simulink model "GFL_phasejump"  (R2022a)
settings: Solver=FixedStepAuto  StartTime=0.0  StopTime=t_end+t_sim_start  FixedStep=Ts  RelTol=1e-3
undefined symbols (not defined in the file or in its folder): Cf, dc_ref, DiscIntNeverNeededParam, dt, Id0, Id_limit, initial, Iq0, ki_pll, ki_v_dc, kp_pll, kp_v_dc, Lc, Lf, Lg1, Lg11, Lgg, m_v, phasejum, Rf, Rg1, Rg11, Rgg, Sbase, t0, t0_jump, t_sim_start, tc, Ts, v_sag, Vac_ref, Vbase, Vdc_ref, w_i_GFL, w_limit, w_pll, w_tau, w_tvc, Wbase, Y_dc, Zbase
libraries: spsVoltageMeasurementLib x41, spsCurrentMeasurementLib x36, spsThreePhaseSeriesRLCBranchLib x14, spsControlledVoltageSourceLib x12, spsSeriesRLCBranchLib x8, spsControlledCurrentSourceLib x4, spsIdealSwitchLib x3, spsThreePhaseBreakerLib x2, spsDCVoltageSourceLib x1, spsThreePhaseParallelRLCBranchLib x1, spsThreePhaseFaultLib x1, spspowerguiLib x1
(part 1 of 3)
settings Model: Creator=admin_user  LastModifiedBy=yz7521
settings SolverCC: AlgebraicLoopSolver=TrustRegion
settings DataIOCC: ReturnWorkspaceOutputs=off
settings DebuggingCC: SFMachineParentedDataDiag=warning
settings RTWCC: DLArmComputeVersion=19.05

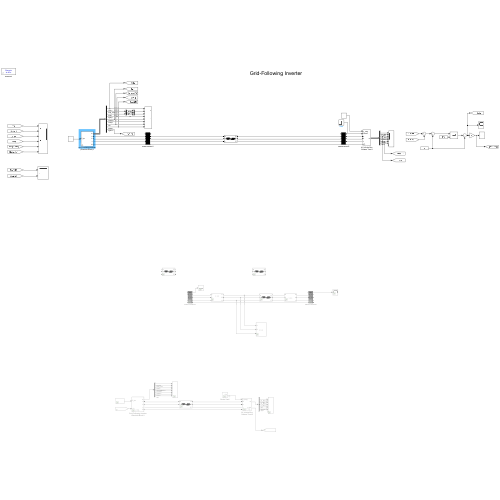
[thumbnail: Simulink's stored preview of the top-level diagram]
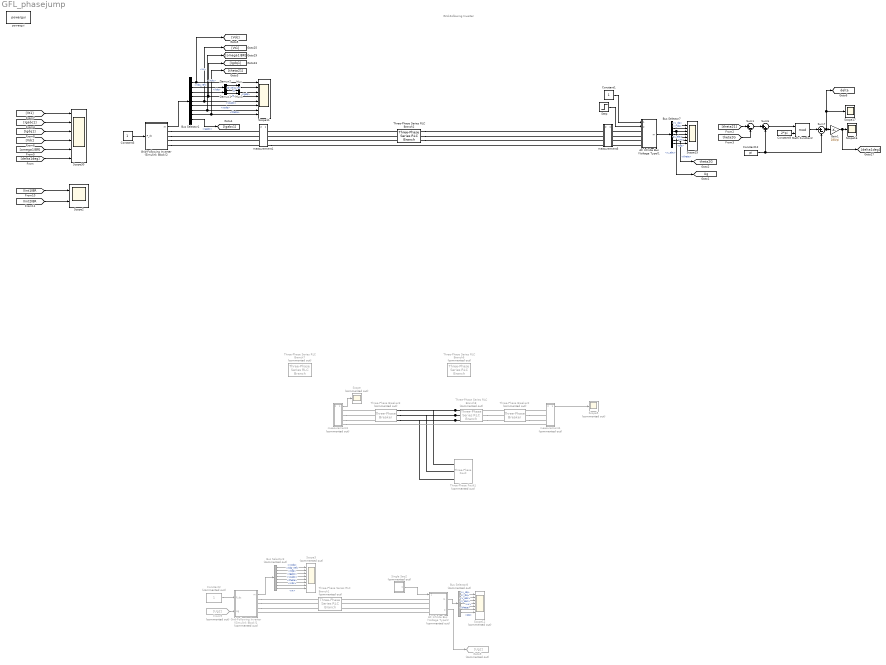
== system GFL_phasejump ==
  note: Grid-Following Inverter
  AC Infinite Bus (Voltage Type)1 : Subsystem  mask{Ts=Ts, Sbase=Sbase, Vbase=Vbase, Wbase=Wbase, theta0=0, w=Wbase, R=1e-30}
      mask prompts: Ts "Ts (s), samping period"; Sbase "Sbase (VA), power base"; Vbase "Vbase (V), voltage base"; Wbase "Wbase (rad/s), frequency base"; theta0 "theta0 (rad), initial angle"; w "w (rad/s), frequency"; R "R (Ohm), resistance"
  AC Infinite Bus (Voltage Type)2 : Subsystem  Commented=on  AncestorBlock=|  mask{Ts=Ts, Sbase=Sbase, Vbase=Vbase, Wbase=Wbase, theta0=0, w=Wbase, R=1e-30}
      | SimplusGT/AC Infinite Bus
      | (Voltage Type)
      mask prompts: Ts "Ts (s), samping period"; Sbase "Sbase (VA), power base"; Vbase "Vbase (V), voltage base"; Wbase "Wbase (rad/s), frequency base"; theta0 "theta0 (rad), initial angle"; w "w (rad/s), frequency"; R "R (Ohm), resistance"
  Bus Selector1 : BusSelector  OutputSignals=Vdc,ildq_ref,ildq,igdq,vcabc,vcdq,w,theta,igabc
  Bus Selector3 : BusSelector  Commented=on  OutputSignals=vcdq,ildq_ref,ildq,igabc,vcabc,theta,Vdc,w
  Bus Selector7 : BusSelector  OutputSignals=v_dq,i_dq,v_abc,i_abc,w,theta,pq
  Bus Selector8 : BusSelector  Commented=on  OutputSignals=v_dq,i_dq,v_abc,i_abc,w,theta,pq
  Constant1 : Constant
  Constant12 : Constant  Value=pi
  Constant2 : Constant  Commented=on
  Constant3 : Constant
  Constant9 : Constant  Value=2*pi
  Demux1 : Demux  Outputs=2
  Demux2 : Demux  Outputs=2
  From9 : From  Commented=on  GotoTag=Ug2
  Gain1 : Gain  Gain=180/pi
  Goto9 : Goto  Commented=on  GotoTag=Ug2
  Grid-Following Inverter (Simulink Block)1 : Subsystem  Commented=on  AncestorBlock=|  mask{Ts=Ts, Sbase=Sbase, Vbase=Vbase, Wbase=Wbase, w_i=w_i_GFL, w_pll=w_pll, w_tau=w_tau, Lf=Lf, Cf=Cf, Lc=Lc}
      | SimplusGT/Grid-Following Inverter
      | (Simulink Block)
      mask prompts: Ts "Ts (s), sampling period"; Sbase "Sbase (VA), base power"; Vbase "Vbase (V), base voltage"; Wbase "Wbase (rad/s), base frequency"; w_i "w_i (rad/s), current-loop bandwidth"; w_pll "w_pll (rad/s), PLL bandwidth"; w_tau "w_tau (rad/s), PLL filter bandwidth"; Lf "Lf (pu), LCL filter"; Cf "Cf (pu), LCL filter"; Lc "Lc (pu), LCL filter"
  Grid-Following Inverter (Simulink Block)2 : Subsystem  mask{Ts=Ts, Sbase=Sbase, Vbase=Vbase, Wbase=Wbase, w_i=w_i_GFL, w_tau=w_tau, Lf=Lf, Cf=Cf, Lc=Lc}
      mask prompts: Ts "Ts (s), sampling period"; Sbase "Sbase (VA), base power"; Vbase "Vbase (V), base voltage"; Wbase "Wbase (rad/s), base frequency"; w_i "w_i (rad/s), current-loop bandwidth"; w_tau "w_tau (rad/s), PLL filter bandwidth"; Lf "Lf (pu), LCL filter"; Cf "Cf (pu), LCL filter"; Lc "Lc (pu), LCL filter"
  Math Function2 : Math  Operator=mod  SignedPower=on
  Mux : Mux  Inputs=2
  Mux1 : Mux  Inputs=2
  Scope : Scope  Commented=on
  Scope11 : Scope  NumInputPorts=8
  Scope12 : Scope  Commented=on  NumInputPorts=8
  Scope15 : Scope  NumInputPorts=8
  Scope16 : Scope
  Scope17 : Scope
  Scope2 : Scope  NumInputPorts=2
  Scope3 : Scope  Commented=on  NumInputPorts=8
  Scope30 : Scope  NumInputPorts=6
  Scope5 : Scope  Commented=on
  Single Sag2 : Subsystem  Commented=on  AncestorBlock=SimplusGT/Single Pulse  mask{t0=t0, dt=dt, Am=v_sag}
      mask prompts: t0 "t0 (s), starting time"; dt "dt (s), pulse width"; Am "Am, pulse amplitude"
  Step : Step  Time=t0_jump  After=phasejum  SampleTime=0
  Sum1 : Sum  Inputs=|+-
  Sum6 : Sum  Inputs=|++
  Sum7 : Sum  Inputs=|+-
  Three-Phase Series RLC Branch1 : spsThreePhaseSeriesRLCBranchLib/Three-Phase Series RLC Branch  Commented=on  LConnTagsString=A|B|C  RConnTagsString=A|B|C  BranchType=RL  Resistance=Rg11*Zbase  Inductance=Lg11*Zbase/Wbase  Capacitance=1/Wbase  Measurements=None
  Three-Phase Series RLC Branch2 : spsThreePhaseSeriesRLCBranchLib/Three-Phase Series RLC Branch  LConnTagsString=A|B|C  RConnTagsString=A|B|C  BranchType=RL  Resistance=Rg11*Zbase  Inductance=Lg11*Zbase/Wbase  Capacitance=1/Wbase  Measurements=None
  Three-Phase Series RLC Branch6 : spsThreePhaseSeriesRLCBranchLib/Three-Phase Series RLC Branch  Commented=on  LConnTagsString=A|B|C  RConnTagsString=A|B|C  BranchType=RL  Resistance=Rgg*Zbase  Inductance=Lgg*Zbase/Wbase  Capacitance=1/Wbase  Measurements=None
  Three-Phase Series RLC Branch7 : spsThreePhaseSeriesRLCBranchLib/Three-Phase Series RLC Branch  Commented=on  LConnTagsString=A|B|C  RConnTagsString=A|B|C  BranchType=RL  Resistance=Rg1*Zbase  Inductance=Lg1*Zbase/Wbase  Capacitance=1/Wbase  Measurements=None
  Three-Phase Series RLC Branch8 : spsThreePhaseSeriesRLCBranchLib/Three-Phase Series RLC Branch  Commented=on  LConnTagsString=A|B|C  RConnTagsString=A|B|C  BranchType=RL  Resistance=Rgg*Zbase  Inductance=Lgg*Zbase/Wbase  Capacitance=1/Wbase  Measurements=None
  Three-Phase Breaker2 : spsThreePhaseBreakerLib/Three-Phase Breaker  Commented=on  InitialState=closed  SwitchA=on  SwitchB=on  SwitchC=on  SwitchTimes=[t0+tc]  External=off  BreakerResistance=0.01e-3  SnubberResistance=1e6  SnubberCapacitance=inf  Measurements=Breaker currents
  Three-Phase Breaker3 : spsThreePhaseBreakerLib/Three-Phase Breaker  Commented=on  InitialState=closed  SwitchA=on  SwitchB=on  SwitchC=on  SwitchTimes=[t0+tc]  External=off  BreakerResistance=0.1e-3  SnubberResistance=1e6  SnubberCapacitance=inf  Measurements=Breaker currents
  Three-Phase Fault1 : spsThreePhaseFaultLib/Three-Phase Fault  Commented=on  InitialStates=0  FaultA=on  FaultB=on  FaultC=on  GroundFault=off  SwitchTimes=[t0]  External=off  SwitchStatus=NaN  FaultResistance=Rf*Zbase  GroundResistance=0.01e-6  SnubberResistance=10e6  SnubberCapacitance=inf  Measurements=None
  measurement1 : Subsystem
      settings: PortSchema="{\"entries\":[{\"content\":{\"sides\":[{\"content\":{\"connectorIds\":[\"Out2\",\"LConn1\",\"LConn2\",\"LConn3\",\"LConn4\"]},\"type\":\"ConnectorPlacement.EquallySpacedRectSide\",\"uuid\":\"b97639c7-89ad-4c11-8fcc-ddc4f61f4533\"},{\"content\":{\"connectorIds\":[\"Out1\",\"RConn1\",\"RConn2\",\"RConn3\",\"RConn4\"],\"side\":\"RIGHT\"},\"type\":\"ConnectorPlacement.EquallySpacedRectSide\",\"uuid\":\"3b8f0759-83d7-4d3a-a5c5-bdf29e7cbe5b\"},{\"content\":{\"connectorIds\":[],\"side\":\"TOP\"},\"type\":\"ConnectorPlacement.EquallySpacedRectSide\",\"uuid\":\"1e391932-f1e1-4127-bfe0-28b7de5de667\"},{\"content\":{\"connectorIds\":[],\"side\":\"BOTTOM\"},\"type\":\"ConnectorPlacement.EquallySpacedRectSide\",\"uuid\":\"f0c236e9-048a-4270-a45f-ff2fecf0ec8b\"}]},\"type\":\"ConnectorPlacement.EquallySpacedConnector\",\"uuid\":\"002609f8-6c16-431f-ae58-b6d94c927972\"}],\"packageUris\":[\"http://schema.mathworks.com/mf0/Connector/R2020b\"],\"version\":\"1.0\"}"
  measurement3 : Subsystem  Commented=on
      settings: PortSchema="{\"entries\":[{\"content\":{\"sides\":[{\"content\":{\"connectorIds\":[\"Out2\",\"LConn1\",\"LConn2\",\"LConn3\",\"LConn4\"]},\"type\":\"ConnectorPlacement.EquallySpacedRectSide\",\"uuid\":\"b97639c7-89ad-4c11-8fcc-ddc4f61f4533\"},{\"content\":{\"connectorIds\":[\"Out1\",\"RConn1\",\"RConn2\",\"RConn3\",\"RConn4\"],\"side\":\"RIGHT\"},\"type\":\"ConnectorPlacement.EquallySpacedRectSide\",\"uuid\":\"3b8f0759-83d7-4d3a-a5c5-bdf29e7cbe5b\"},{\"content\":{\"connectorIds\":[],\"side\":\"TOP\"},\"type\":\"ConnectorPlacement.EquallySpacedRectSide\",\"uuid\":\"1e391932-f1e1-4127-bfe0-28b7de5de667\"},{\"content\":{\"connectorIds\":[],\"side\":\"BOTTOM\"},\"type\":\"ConnectorPlacement.EquallySpacedRectSide\",\"uuid\":\"f0c236e9-048a-4270-a45f-ff2fecf0ec8b\"}]},\"type\":\"ConnectorPlacement.EquallySpacedConnector\",\"uuid\":\"002609f8-6c16-431f-ae58-b6d94c927972\"}],\"packageUris\":[\"http://schema.mathworks.com/mf0/Connector/R2020b\"],\"version\":\"1.0\"}"
  measurement4 : Subsystem  Commented=on
      settings: PortSchema="{\"entries\":[{\"content\":{\"sides\":[{\"content\":{\"connectorIds\":[\"Out2\",\"LConn1\",\"LConn2\",\"LConn3\",\"LConn4\"]},\"type\":\"ConnectorPlacement.EquallySpacedRectSide\",\"uuid\":\"b97639c7-89ad-4c11-8fcc-ddc4f61f4533\"},{\"content\":{\"connectorIds\":[\"Out1\",\"RConn1\",\"RConn2\",\"RConn3\",\"RConn4\"],\"side\":\"RIGHT\"},\"type\":\"ConnectorPlacement.EquallySpacedRectSide\",\"uuid\":\"3b8f0759-83d7-4d3a-a5c5-bdf29e7cbe5b\"},{\"content\":{\"connectorIds\":[],\"side\":\"TOP\"},\"type\":\"ConnectorPlacement.EquallySpacedRectSide\",\"uuid\":\"1e391932-f1e1-4127-bfe0-28b7de5de667\"},{\"content\":{\"connectorIds\":[],\"side\":\"BOTTOM\"},\"type\":\"ConnectorPlacement.EquallySpacedRectSide\",\"uuid\":\"f0c236e9-048a-4270-a45f-ff2fecf0ec8b\"}]},\"type\":\"ConnectorPlacement.EquallySpacedConnector\",\"uuid\":\"002609f8-6c16-431f-ae58-b6d94c927972\"}],\"packageUris\":[\"http://schema.mathworks.com/mf0/Connector/R2020b\"],\"version\":\"1.0\"}"
  measurement5 : Subsystem
      settings: PortSchema="{\"entries\":[{\"content\":{\"sides\":[{\"content\":{\"connectorIds\":[\"Out2\",\"LConn1\",\"LConn2\",\"LConn3\",\"LConn4\"]},\"type\":\"ConnectorPlacement.EquallySpacedRectSide\",\"uuid\":\"b97639c7-89ad-4c11-8fcc-ddc4f61f4533\"},{\"content\":{\"connectorIds\":[\"Out1\",\"RConn1\",\"RConn2\",\"RConn3\",\"RConn4\"],\"side\":\"RIGHT\"},\"type\":\"ConnectorPlacement.EquallySpacedRectSide\",\"uuid\":\"3b8f0759-83d7-4d3a-a5c5-bdf29e7cbe5b\"},{\"content\":{\"connectorIds\":[],\"side\":\"TOP\"},\"type\":\"ConnectorPlacement.EquallySpacedRectSide\",\"uuid\":\"1e391932-f1e1-4127-bfe0-28b7de5de667\"},{\"content\":{\"connectorIds\":[],\"side\":\"BOTTOM\"},\"type\":\"ConnectorPlacement.EquallySpacedRectSide\",\"uuid\":\"f0c236e9-048a-4270-a45f-ff2fecf0ec8b\"}]},\"type\":\"ConnectorPlacement.EquallySpacedConnector\",\"uuid\":\"002609f8-6c16-431f-ae58-b6d94c927972\"}],\"packageUris\":[\"http://schema.mathworks.com/mf0/Connector/R2020b\"],\"version\":\"1.0\"}"
  powergui : spspowerguiLib/powergui  Priority=1  SimulationMode=Discrete  SampleTime=Ts  frequency=60  Iterations=50  frequencyindice=0  Pbase=100e6  ErrMax=1e-4  UnitsV=kV  UnitsW=MW  buscounter=0  FunctionMessages=off  echomessages=off  EnableUseOfTLC=off  CurrentSourceSwitches=off  DisableSnubberDevices=off  DisableRonSwitches=off  DisableVfSwitches=off  DisplayEquations=off  AutomaticDiscreteSolvers=off  SolverType=Tustin/Backward Euler (TBE)  Interpol=off  ExternalGateDelay=off  methode=off  Ts=100  x0status=blocks  SPID=on  SwTol=0  HookPort=off  NonlinearTolerance=1e-4  nMaxIteration=100  ContinueOnMaxIteration=off  RestoreLinks=warning  ResistiveCurrentMeasurement=off  Frange=[0:2:500]  Ylog=off  Xlog=on  ShowGrid=off  save=off  variable=ZData  structure=0  ZoomFFT=off  StartTime=0.0  cycles=1  DisplayStyle=1  fundamental=60  FreqAxis=off  MaxFrequency=1000  frequencyindicesteady=1  RmsSteady=1  display=off
  tag scope: Ug=global, delta=global, theta2G=global
  wires:
  [theta21] -> Sum1/1
  Grid-Following Inverter (Simulink Block)2/1(m) -> Bus Selector1/1
  Constant12/1 -> Sum6/2, Sum7/2
  Sum1/1 -> Sum6/1
  Bus Selector7/3 -> [Ug], Scope15/3  "<v_abc>"
  AC Infinite Bus (Voltage Type)1/1(m) -> Bus Selector7/1
  Constant9/1 -> Math Function2/2
  [theta2G] -> Sum1/2
  Gain1/1 -> [delta1deg], Scope16/1
  Bus Selector7/4 -> Scope15/4  "<i_abc>"
  Bus Selector7/5 -> Scope15/5  "<w>"
  Sum7/1 -> [delta], Scope17/1, Gain1/1
  Sum6/1 -> Math Function2/1
  Math Function2/1 -> Sum7/1
  Bus Selector7/7 -> Scope15/7  "<pq>"
  Bus Selector7/6 -> [theta2G], Scope15/6  "<theta>"
  Bus Selector7/1 -> Scope15/1  "<v_dq>"
  Step/1 -> AC Infinite Bus (Voltage Type)1/2(Phase)
  Bus Selector7/2 -> Scope15/2  "<i_dq>"
  [Vt1] -> Scope30/1
  measurement3/1(Iabc) -> Scope/1
  measurement4/1(Iabc) -> Scope5/1
  Bus Selector1/1 -> Scope11/1, [Vdc]  "<Vdc>"
  Bus Selector1/4 -> Scope11/4, [Igdq1]  "<igdq>"
  Bus Selector1/5 -> Scope11/5, [Vt1]  "<vcabc>"
  Bus Selector1/7 -> Scope11/7, [omega1IBR]  "<w>"
  Bus Selector1/8 -> Scope11/8, [theta21]  "<theta>"
  Bus Selector1/9 -> [Igabc1]  "<igabc>"
  [Igabc1] -> Scope30/2
  [Igdq1] -> Scope30/3
  [delta1deg] -> Scope30/6
  [omega1IBR] -> Scope30/5
  [Vdc] -> Scope30/4
  Single Sag2/1(Out) -> AC Infinite Bus (Voltage Type)2/1(v_mag)
  Constant2/1 -> Grid-Following Inverter (Simulink Block)1/1(P_dc)
  Bus Selector8/3 -> Scope12/3  "<v_abc>"
  Bus Selector3/3 -> Scope3/3  "<ildq>"
  Bus Selector3/5 -> Scope3/5  "<vcabc>"
  Bus Selector8/6 -> Scope12/6  "<theta>"
  Bus Selector8/7 -> Scope12/7  "<pq>"
  Bus Selector3/8 -> Scope3/8  "<w>"
  From9/1 -> Grid-Following Inverter (Simulink Block)1/2(Ug)
  Bus Selector8/4 -> Scope12/4  "<i_abc>"
  Bus Selector3/7 -> Scope3/7  "<Vdc>"
  Grid-Following Inverter (Simulink Block)1/1(m) -> Bus Selector3/1
  Bus Selector3/4 -> Scope3/4  "<igabc>"
  Bus Selector8/5 -> Scope12/5  "<w>"
  Bus Selector8/1 -> Scope12/1  "<v_dq>"
  AC Infinite Bus (Voltage Type)2/1(m) -> Bus Selector8/1
  AC Infinite Bus (Voltage Type)2/2(v_abc) -> Goto9/1
  Bus Selector3/6 -> Scope3/6  "<theta>"
  Bus Selector8/2 -> Scope12/2  "<i_dq>"
  Bus Selector3/1 -> Scope3/1  "<vcdq>"
  Bus Selector3/2 -> Scope3/2  "<ildq_ref>"
  Bus Selector1/2 -> Demux2/1  "<ildq_ref>"
  Bus Selector1/3 -> Demux1/1  "<ildq>"
  Demux2/1 -> Mux/1  "Id_ref"
  Demux1/1 -> Mux/2  "Id"
  Demux2/2 -> Mux1/1  "Iq_ref"
  Demux1/2 -> Mux1/2  "Iq"
  Mux/1 -> Scope11/2
  Mux1/1 -> Scope11/3
  Bus Selector1/6 -> Scope11/6  "<vcdq>"
  Constant1/1 -> AC Infinite Bus (Voltage Type)1/1(v_mag)
  Constant3/1 -> Grid-Following Inverter (Simulink Block)2/1(P_dc)
  [Xint1IBR] -> Scope2/1
  [Xint2IBR] -> Scope2/2
  connections:
  Grid-Following Inverter (Simulink Block)2/RConn1 -- measurement1/LConn1
  Grid-Following Inverter (Simulink Block)2/RConn2 -- measurement1/LConn2
  Grid-Following Inverter (Simulink Block)2/RConn4 -- measurement1/LConn4
  measurement1/RConn4 -- measurement5/LConn4
  AC Infinite Bus (Voltage Type)1/LConn4 -- measurement5/RConn4
  AC Infinite Bus (Voltage Type)1/LConn1 -- measurement5/RConn1
  AC Infinite Bus (Voltage Type)1/LConn2 -- measurement5/RConn2
  AC Infinite Bus (Voltage Type)1/LConn3 -- measurement5/RConn3
  Three-Phase Series RLC Branch2/LConn1 -- measurement5/LConn1
  Three-Phase Series RLC Branch2/LConn2 -- measurement5/LConn2
  Three-Phase Series RLC Branch2/LConn3 -- measurement5/LConn3
  Three-Phase Series RLC Branch2/RConn3 -- measurement1/RConn3
  Three-Phase Series RLC Branch2/RConn2 -- measurement1/RConn2
  Three-Phase Series RLC Branch2/RConn1 -- measurement1/RConn1
  Three-Phase Series RLC Branch8/RConn1 -- Three-Phase Fault1/LConn1 -- Three-Phase Breaker3/LConn3
  Three-Phase Series RLC Branch8/RConn3 -- Three-Phase Fault1/LConn3 -- Three-Phase Breaker3/LConn1
  Three-Phase Series RLC Branch8/RConn2 -- Three-Phase Fault1/LConn2 -- Three-Phase Breaker3/LConn2
  measurement3/RConn2 -- Three-Phase Breaker3/RConn2
  Three-Phase Breaker2/RConn2 -- measurement4/LConn2
  measurement3/RConn3 -- Three-Phase Breaker3/RConn1
  Three-Phase Series RLC Branch8/LConn3 -- Three-Phase Breaker2/LConn3
  Three-Phase Breaker2/RConn3 -- measurement4/LConn3
  Three-Phase Breaker3/RConn3 -- measurement3/RConn1
  Three-Phase Breaker2/LConn1 -- Three-Phase Series RLC Branch8/LConn1
  measurement4/LConn1 -- Three-Phase Breaker2/RConn1
  measurement3/RConn4 -- measurement4/LConn4
  Three-Phase Series RLC Branch8/LConn2 -- Three-Phase Breaker2/LConn2
  Grid-Following Inverter (Simulink Block)1/RConn3 -- Three-Phase Series RLC Branch1/RConn3
  AC Infinite Bus (Voltage Type)2/LConn4 -- Grid-Following Inverter (Simulink Block)1/RConn4
  Grid-Following Inverter (Simulink Block)1/RConn1 -- Three-Phase Series RLC Branch1/RConn1
  AC Infinite Bus (Voltage Type)2/LConn2 -- Three-Phase Series RLC Branch1/LConn2
  AC Infinite Bus (Voltage Type)2/LConn3 -- Three-Phase Series RLC Branch1/LConn3
  Grid-Following Inverter (Simulink Block)1/RConn2 -- Three-Phase Series RLC Branch1/RConn2
  AC Infinite Bus (Voltage Type)2/LConn1 -- Three-Phase Series RLC Branch1/LConn1
  Grid-Following Inverter (Simulink Block)2/RConn3 -- measurement1/LConn3

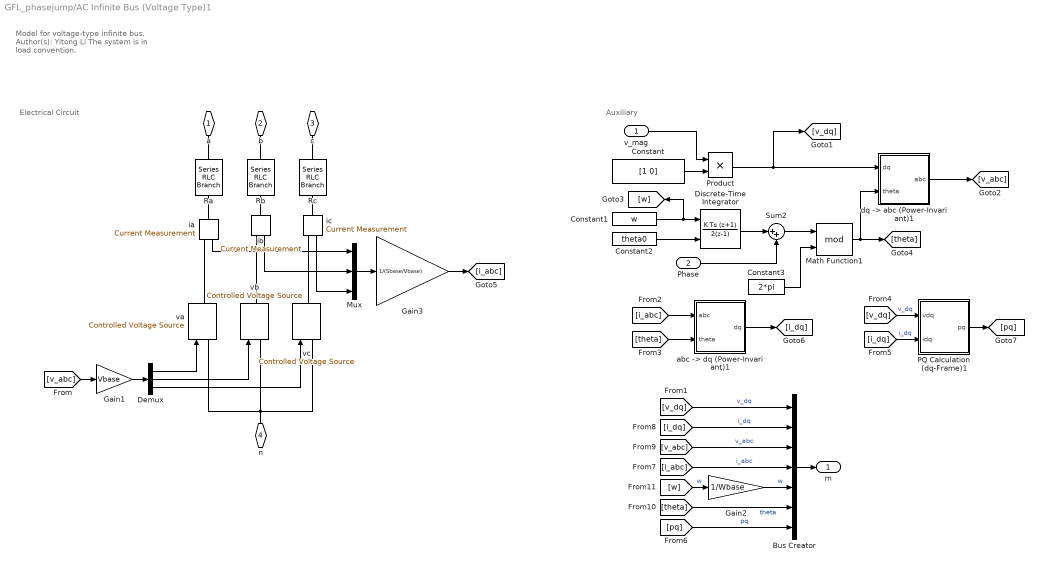
== system GFL_phasejump/AC Infinite Bus (Voltage Type)1 ==
  note: Auxiliary
  note: Electrical Circuit
  note: Model for voltage-type infinite bus.
      |
      | Author(s): Yitong Li
      |
      | The system is in load convention.
  v_mag : Inport
  Phase : Inport  Port=2
  Bus Creator : BusCreator  Inputs=7
  Constant : Constant  Value=[1 0]
  Constant1 : Constant  Value=w
  Constant2 : Constant  Value=theta0
  Constant3 : Constant  Value=2*pi
  Demux : Demux  Outputs=3
  Discrete-Time Integrator : DiscreteIntegrator  IntegratorMethod=Integration: Trapezoidal  InitialConditionSource=external  SampleTime=-1  ICPrevOutput=DiscIntNeverNeededParam  ICPrevScaledInput=DiscIntNeverNeededParam
  Gain1 : Gain  Gain=Vbase
  Gain2 : Gain  Gain=1/Wbase
  Gain3 : Gain  Gain=1/(Sbase/Vbase)
  Math Function1 : Math  Operator=mod  SignedPower=on
  Mux : Mux  Inputs=3
  PQ Calculation (dq-Frame)1 : Subsystem  AncestorBlock=|
      | SimplusGT/PQ Calculation
      | (dq-Frame)
  Product : Product
  Ra : spsSeriesRLCBranchLib/Series RLC Branch  LConnTagsString=__new0  RConnTagsString=__new0  BranchType=R  Resistance=R  Inductance=1e-3  SetiL0=off  InitialCurrent=0  Capacitance=1e-6  Setx0=off  InitialVoltage=0  Measurements=None
  Rb : spsSeriesRLCBranchLib/Series RLC Branch  LConnTagsString=__new0  RConnTagsString=__new0  BranchType=R  Resistance=R  Inductance=1e-3  SetiL0=off  InitialCurrent=0  Capacitance=1e-6  Setx0=off  InitialVoltage=0  Measurements=None
  Rc : spsSeriesRLCBranchLib/Series RLC Branch  LConnTagsString=__new0  RConnTagsString=__new0  BranchType=R  Resistance=R  Inductance=1e-3  SetiL0=off  InitialCurrent=0  Capacitance=1e-6  Setx0=off  InitialVoltage=0  Measurements=None
  Sum2 : Sum  Inputs=|++
  "abc -> dq (Power-Invariant)1" : Subsystem  AncestorBlock=|
      | SimplusGT/abc -> dq
      | (Power-Invariant)
  "dq -> abc (Power-Invariant)1" : Subsystem  AncestorBlock=|
      | SimplusGT/dq -> abc
      | (Power-Invariant)
  ia : spsCurrentMeasurementLib/Current Measurement  PhasorSimulation=off  OutputType=Complex  PSBequivalent=0
  ib : spsCurrentMeasurementLib/Current Measurement  PhasorSimulation=off  OutputType=Complex  PSBequivalent=0
  ic : spsCurrentMeasurementLib/Current Measurement  PhasorSimulation=off  OutputType=Complex  PSBequivalent=0
  va : spsControlledVoltageSourceLib/Controlled Voltage Source  Initialize=on  Source_Type=AC  Amplitude=0  Phase=0  Frequency=0  Measurements=None
  vb : spsControlledVoltageSourceLib/Controlled Voltage Source  Initialize=on  Source_Type=AC  Amplitude=0  Phase=0  Frequency=0  Measurements=None
  vc : spsControlledVoltageSourceLib/Controlled Voltage Source  Initialize=on  Source_Type=AC  Amplitude=0  Phase=0  Frequency=0  Measurements=None
  a : PMIOPort  Side=Left
  b : PMIOPort  Port=2  Side=Left
  c : PMIOPort  Port=3  Side=Left
  n : PMIOPort  Port=4  Side=Left
  m : Outport
  wires:
  [pq] -> Bus Creator/7  "pq"
  PQ Calculation (dq-Frame)1/1(pq) -> [pq]
  [i_dq] -> PQ Calculation (dq-Frame)1/2(idq)  "i_dq"
  [v_dq] -> PQ Calculation (dq-Frame)1/1(vdq)  "v_dq"
  Gain3/1 -> [i_abc]
  Mux/1 -> Gain3/1
  Gain1/1 -> Demux/1
  "abc -> dq (Power-Invariant)1"/1(dq) -> [i_dq]
  [theta] -> "abc -> dq (Power-Invariant)1"/2(theta)
  [i_abc] -> "abc -> dq (Power-Invariant)1"/1(abc)
  ic/1 -> Mux/3
  ib/1 -> Mux/2
  ia/1 -> Mux/1
  [theta] -> Bus Creator/6  "theta"
  Bus Creator/1 -> m/1
  [i_dq] -> Bus Creator/2  "i_dq"
  Gain2/1 -> Bus Creator/5  "w"
  [v_abc] -> Bus Creator/3  "v_abc"
  [w] -> Gain2/1  "w"
  [i_abc] -> Bus Creator/4  "i_abc"
  [v_dq] -> Bus Creator/1  "v_dq"
  Constant3/1 -> Math Function1/2
  "dq -> abc (Power-Invariant)1"/1(abc) -> [v_abc]
  Constant1/1 -> [w], Discrete-Time Integrator/1
  Constant2/1 -> Discrete-Time Integrator/2
  Math Function1/1 -> [theta], "dq -> abc (Power-Invariant)1"/2(theta)
  Demux/3 -> vc/1
  Demux/2 -> vb/1
  Demux/1 -> va/1
  [v_abc] -> Gain1/1
  Constant/1 -> Product/2
  v_mag/1 -> Product/1
  Product/1 -> [v_dq], "dq -> abc (Power-Invariant)1"/1(dq)
  Discrete-Time Integrator/1 -> Sum2/1
  Sum2/1 -> Math Function1/1
  Phase/1 -> Sum2/2
  connections:
  Rc/LConn1 -- c/RConn1
  Rc/RConn1 -- ic/LConn1
  Rb/LConn1 -- b/RConn1
  ib/LConn1 -- Rb/RConn1
  Ra/LConn1 -- a/RConn1
  Ra/RConn1 -- ia/LConn1
  ic/RConn1 -- vc/RConn1
  ib/RConn1 -- vb/RConn1
  ia/RConn1 -- va/RConn1
  vb/LConn1 -- va/LConn1 -- n/RConn1 -- vc/LConn1

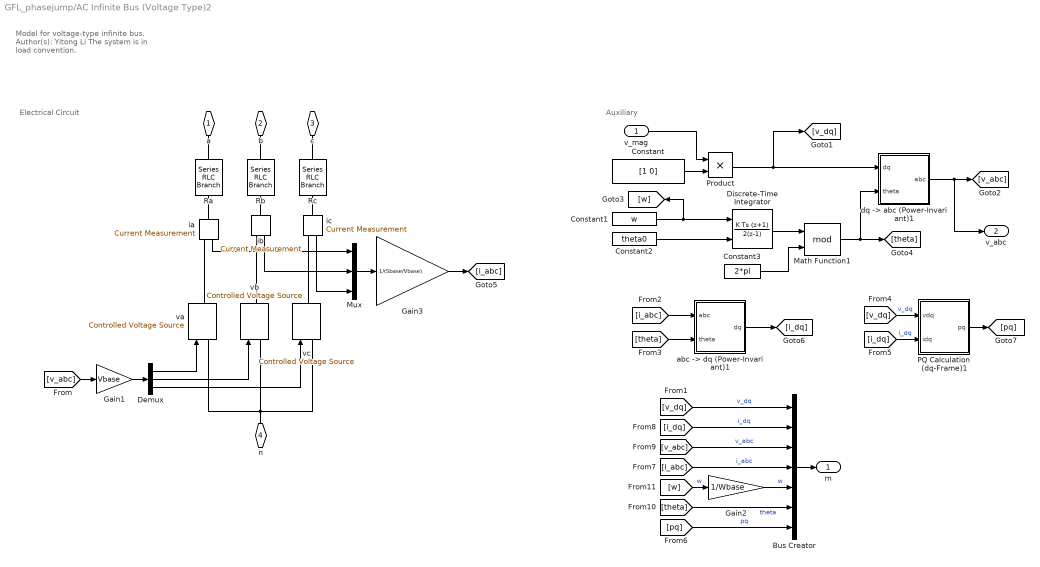
== system GFL_phasejump/AC Infinite Bus (Voltage Type)2 ==
  note: Auxiliary
  note: Electrical Circuit
  note: Model for voltage-type infinite bus.
      |
      | Author(s): Yitong Li
      |
      | The system is in load convention.
  v_mag : Inport
  Bus Creator : BusCreator  Inputs=7
  Constant : Constant  Value=[1 0]
  Constant1 : Constant  Value=w
  Constant2 : Constant  Value=theta0
  Constant3 : Constant  Value=2*pi
  Demux : Demux  Outputs=3
  Discrete-Time Integrator : DiscreteIntegrator  IntegratorMethod=Integration: Trapezoidal  InitialConditionSource=external  SampleTime=-1  ICPrevOutput=DiscIntNeverNeededParam  ICPrevScaledInput=DiscIntNeverNeededParam
  Gain1 : Gain  Gain=Vbase
  Gain2 : Gain  Gain=1/Wbase
  Gain3 : Gain  Gain=1/(Sbase/Vbase)
  Math Function1 : Math  Operator=mod  SignedPower=on
  Mux : Mux  Inputs=3
  PQ Calculation (dq-Frame)1 : Subsystem  AncestorBlock=|
      | SimplusGT/PQ Calculation
      | (dq-Frame)
  Product : Product
  Ra : spsSeriesRLCBranchLib/Series RLC Branch  LConnTagsString=__new0  RConnTagsString=__new0  BranchType=R  Resistance=R  Inductance=1e-3  SetiL0=off  InitialCurrent=0  Capacitance=1e-6  Setx0=off  InitialVoltage=0  Measurements=None
  Rb : spsSeriesRLCBranchLib/Series RLC Branch  LConnTagsString=__new0  RConnTagsString=__new0  BranchType=R  Resistance=R  Inductance=1e-3  SetiL0=off  InitialCurrent=0  Capacitance=1e-6  Setx0=off  InitialVoltage=0  Measurements=None
  Rc : spsSeriesRLCBranchLib/Series RLC Branch  LConnTagsString=__new0  RConnTagsString=__new0  BranchType=R  Resistance=R  Inductance=1e-3  SetiL0=off  InitialCurrent=0  Capacitance=1e-6  Setx0=off  InitialVoltage=0  Measurements=None
  "abc -> dq (Power-Invariant)1" : Subsystem  AncestorBlock=|
      | SimplusGT/abc -> dq
      | (Power-Invariant)
  "dq -> abc (Power-Invariant)1" : Subsystem  AncestorBlock=|
      | SimplusGT/dq -> abc
      | (Power-Invariant)
  ia : spsCurrentMeasurementLib/Current Measurement  PhasorSimulation=off  OutputType=Complex  PSBequivalent=0
  ib : spsCurrentMeasurementLib/Current Measurement  PhasorSimulation=off  OutputType=Complex  PSBequivalent=0
  ic : spsCurrentMeasurementLib/Current Measurement  PhasorSimulation=off  OutputType=Complex  PSBequivalent=0
  va : spsControlledVoltageSourceLib/Controlled Voltage Source  Initialize=on  Source_Type=AC  Amplitude=0  Phase=0  Frequency=0  Measurements=None
  vb : spsControlledVoltageSourceLib/Controlled Voltage Source  Initialize=on  Source_Type=AC  Amplitude=0  Phase=0  Frequency=0  Measurements=None
  vc : spsControlledVoltageSourceLib/Controlled Voltage Source  Initialize=on  Source_Type=AC  Amplitude=0  Phase=0  Frequency=0  Measurements=None
  a : PMIOPort  Side=Left
  b : PMIOPort  Port=2  Side=Left
  c : PMIOPort  Port=3  Side=Left
  n : PMIOPort  Port=4  Side=Left
  m : Outport
  v_abc : Outport  Port=2
  wires:
  [pq] -> Bus Creator/7  "pq"
  PQ Calculation (dq-Frame)1/1(pq) -> [pq]
  [i_dq] -> PQ Calculation (dq-Frame)1/2(idq)  "i_dq"
  [v_dq] -> PQ Calculation (dq-Frame)1/1(vdq)  "v_dq"
  Gain3/1 -> [i_abc]
  Mux/1 -> Gain3/1
  Gain1/1 -> Demux/1
  "abc -> dq (Power-Invariant)1"/1(dq) -> [i_dq]
  [theta] -> "abc -> dq (Power-Invariant)1"/2(theta)
  [i_abc] -> "abc -> dq (Power-Invariant)1"/1(abc)
  ic/1 -> Mux/3
  ib/1 -> Mux/2
  ia/1 -> Mux/1
  [theta] -> Bus Creator/6  "theta"
  Bus Creator/1 -> m/1
  [i_dq] -> Bus Creator/2  "i_dq"
  Gain2/1 -> Bus Creator/5  "w"
  [v_abc] -> Bus Creator/3  "v_abc"
  [w] -> Gain2/1  "w"
  [i_abc] -> Bus Creator/4  "i_abc"
  [v_dq] -> Bus Creator/1  "v_dq"
  Discrete-Time Integrator/1 -> Math Function1/1
  Constant3/1 -> Math Function1/2
  "dq -> abc (Power-Invariant)1"/1(abc) -> v_abc/1, [v_abc]
  Constant1/1 -> [w], Discrete-Time Integrator/1
  Constant2/1 -> Discrete-Time Integrator/2
  Math Function1/1 -> [theta], "dq -> abc (Power-Invariant)1"/2(theta)
  Demux/3 -> vc/1
  Demux/2 -> vb/1
  Demux/1 -> va/1
  [v_abc] -> Gain1/1
  Constant/1 -> Product/2
  v_mag/1 -> Product/1
  Product/1 -> [v_dq], "dq -> abc (Power-Invariant)1"/1(dq)
  connections:
  Rc/LConn1 -- c/RConn1
  Rc/RConn1 -- ic/LConn1
  Rb/LConn1 -- b/RConn1
  ib/LConn1 -- Rb/RConn1
  Ra/LConn1 -- a/RConn1
  Ra/RConn1 -- ia/LConn1
  ic/RConn1 -- vc/RConn1
  ib/RConn1 -- vb/RConn1
  ia/RConn1 -- va/RConn1
  vb/LConn1 -- va/LConn1 -- n/RConn1 -- vc/LConn1

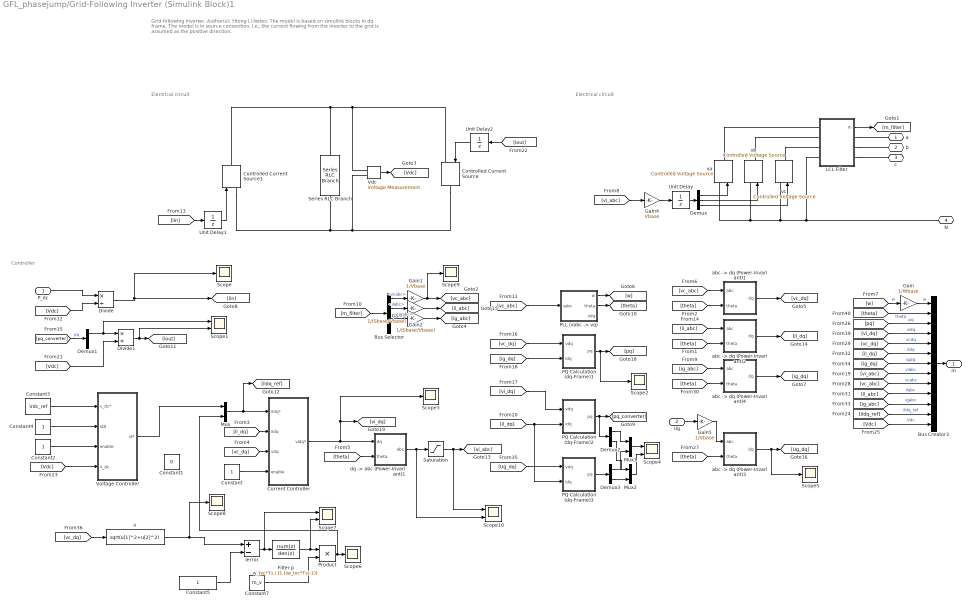
== system GFL_phasejump/Grid-Following Inverter (Simulink Block)1 ==
  note: Electrical circuit
  note: Controller
  note: Electrical circuit
  note: Grid-following inverter.
      |
      | Author(s): Yitong Li
      |
      | Notes:
      |
      | The model is based on simulink blocks in dq frame.
      |
      | The model is in source convention, i.e., the current flowing from the inverter to the grid is assumed as the positive direction.
  P_dc : Inport
  Ug : Inport  Port=2
  Bus Creator3 : BusCreator  Inputs=13
  Bus Selector : BusSelector  OutputSignals=vcabc,ilabc,igabc,viiabc
  Constant{,2,4..5} (4 alike) : Constant
  Constant1 : Constant  Value=0
  Constant3 : Constant  Value=Vdc_ref
  Constant7 : Constant  Value=m_v
  Controlled Current Source : spsControlledCurrentSourceLib/Controlled Current Source  Initialize=on  Source_Type=AC  Amplitude=0  Phase=0  Frequency=0  Measurements=None
  Controlled Current Source1 : spsControlledCurrentSourceLib/Controlled Current Source  Initialize=on  Source_Type=AC  Amplitude=0  Phase=0  Frequency=0  Measurements=None
  Current Controller : Subsystem  mask{Ts=Ts, Wbase=Wbase, Lf=Lf/Wbase, Kg=0, Kp=w_i*Lf/Wbase, Ki=w_i*w_i/4*Lf/Wbase, vdmax=inf, vqmax=inf, Kcd=0}
      mask prompts: Ts "Sampling Time (s)"; Wbase "Base Angular Frequency (rad/s)"; Lf "Inductance"; Kg "Estimator Gain"; Kp "Proportional Gain"; Ki "Integral Gain"; vdmax "Voltage D Limit"; vqmax "Voltage Q Limit"; Kcd "Cross Decoupling Gain"
  Demux : Demux  Outputs=3
  Demux1 : Demux  Outputs=2
  Demux2 : Demux  Outputs=2
  Demux3 : Demux  Outputs=2
  Divide : Product  Inputs=*/
  Divide1 : Product  Inputs=*/
  Filter p : DiscreteTransferFcn  Numerator=w_tvc*Ts  Denominator=[1 ((w_tvc*Ts)-1)]  SampleTime=Ts
  Gain : Gain  Gain=1/Wbase
  Gain1 : Gain  Gain=1/Vbase
  Gain2 : Gain  Gain=1/(Sbase/Vbase)
  Gain3 : Gain  Gain=1/(Sbase/Vbase)
  Gain4 : Gain  Gain=Vbase
  Gain5 : Gain  Gain=1/Vbase
  Ierror : Sum  Inputs=+-
  LCL Filter : Subsystem  AncestorBlock=SimplexPS/LCL Filter  mask{Lf=Lf*(Vbase^2/Sbase)/Wbase, Rf=Lf*(Vbase^2/Sbase)*1e-3, Lc=Lc*(Vbase^2/Sbase)/Wbase, Rc=Lc*(Vbase^2/Sbase)*2e-2, Cf=Cf*(Sbase/Vbase^2)/Wbase, Rd=1e-5*(Vbase^2/Sbase)}
      mask prompts: Lf "Lf (H)"; Rf "Rf (Ohm)"; Lc "Lc (H)"; Rc "Rc (Ohm)"; Cf "Cf (F)"; Rd "Rd (Ohm)"
  Mux : Mux  Inputs=2
  Mux1 : Mux  Inputs=2
  Mux2 : Mux  Inputs=2
  "PLL (vabc -> vq)" : Subsystem  AncestorBlock=|  mask{Ts=Ts, Vbase=Vbase, Wbase=Wbase, kp=kp_pll, ki=ki_pll, w_tau=w_tau, theta0=0}
      | SimplusGT/PLL
      | (vabc -> vq)
      mask prompts: Ts "Ts (s), sampling period"; Vbase "Vbase (V), base voltage"; Wbase "Wbase (rad/s), base angular frequency"; kp "PLL Proportional Gain"; ki "PLL Integral Gain"; w_tau "w_tau (rad/s), low-pass filter bandwidth"; theta0 "theta0 (rad), initial angle"
  PQ Calculation (dq-Frame)1 : Subsystem  AncestorBlock=|
      | SimplusGT/PQ Calculation
      | (dq-Frame)
  PQ Calculation (dq-Frame)2 : Subsystem  AncestorBlock=|
      | SimplusGT/PQ Calculation
      | (dq-Frame)
  PQ Calculation (dq-Frame)3 : Subsystem  AncestorBlock=|
      | SimplusGT/PQ Calculation
      | (dq-Frame)
  Product : Product
  Saturation : Saturate  UpperLimit=5*sqrt(3/2)  LowerLimit=-5*sqrt(3/2)
  Scope{,2..3,5..6,8..9} (7 alike) : Scope
  Scope{1,4,7,10} (4 alike) : Scope  NumInputPorts=2
  Series RLC Branch : spsSeriesRLCBranchLib/Series RLC Branch  LConnTagsString=__new0  RConnTagsString=__new0  BranchType=RC  Resistance=1e-5*(Vbase^2/Sbase)  Inductance=1e-3  SetiL0=off  InitialCurrent=0  Capacitance=Y_dc*(Sbase/Vbase^2)/Wbase  Setx0=on  InitialVoltage=Vdc_ref  Measurements=None
  Unit Delay : UnitDelay  SampleTime=-1  HasFrameUpgradeWarning=on
  Unit Delay1 : UnitDelay  SampleTime=-1  HasFrameUpgradeWarning=on
  Unit Delay2 : UnitDelay  SampleTime=-1  HasFrameUpgradeWarning=on
  Vdc : spsVoltageMeasurementLib/Voltage Measurement  PhasorSimulation=off  OutputType=Complex  PSBequivalent=0
  Voltage Controller : Subsystem  mask{Ts=Ts, Kp=kp_v_dc*5, Ki=ki_v_dc*5, max=2*sqrt(3/2)}
      mask prompts: Ts "Sampling Time (s)"; Kp "Proportional Gain"; Ki "Integral Gain"; max "Output Limit"
  "abc -> dq (Power-Invariant)1" : Subsystem  AncestorBlock=|
      | SimplusGT/abc -> dq
      | (Power-Invariant)
  "abc -> dq (Power-Invariant)2" : Subsystem  AncestorBlock=|
      | SimplusGT/abc -> dq
      | (Power-Invariant)
  "abc -> dq (Power-Invariant)3" : Subsystem  AncestorBlock=|
      | SimplusGT/abc -> dq
      | (Power-Invariant)
  "abc -> dq (Power-Invariant)4" : Subsystem  AncestorBlock=|
      | SimplusGT/abc -> dq
      | (Power-Invariant)
  "dq -> abc (Power-Invariant)1" : Subsystem  AncestorBlock=|
      | SimplusGT/dq -> abc
      | (Power-Invariant)
  u : Fcn  Expr=sqrt(u[1]^2+u[2]^2)
  va : spsControlledVoltageSourceLib/Controlled Voltage Source  Initialize=on  Source_Type=AC  Amplitude=0  Phase=0  Frequency=0  Measurements=None
  vb : spsControlledVoltageSourceLib/Controlled Voltage Source  Initialize=on  Source_Type=AC  Amplitude=0  Phase=0  Frequency=0  Measurements=None
  vc : spsControlledVoltageSourceLib/Controlled Voltage Source  Initialize=on  Source_Type=AC  Amplitude=0  Phase=0  Frequency=0  Measurements=None
  a : PMIOPort  Side=Right
  b : PMIOPort  Port=2  Side=Right
  c : PMIOPort  Port=3  Side=Right
  N : PMIOPort  Port=4  Side=Right
  m : Outport
  wires:
  [vi_abc] -> Gain4/1
  Gain4/1 -> Unit Delay/1
  Gain3/1 -> [ig_abc]
  Gain2/1 -> [il_abc]
  Gain1/1 -> Scope9/1, [vc_abc]
  [ig_abc] -> Bus Creator3/11  "igabc"
  [il_abc] -> Bus Creator3/10  "ilabc"
  [vc_abc] -> Bus Creator3/9  "vcabc"
  [vi_abc] -> Bus Creator3/8  "viabc"
  [ig_dq] -> Bus Creator3/7  "igdq"
  [il_dq] -> Bus Creator3/6  "ildq"
  [vc_dq] -> Bus Creator3/5  "vcdq"
  [vi_dq] -> Bus Creator3/4  "vidq"
  [pq] -> Bus Creator3/3  "pq"
  [theta] -> Bus Creator3/2  "theta"
  Gain/1 -> Bus Creator3/1  "w"
  [w] -> Gain/1  "w"
  Bus Selector/1 -> Gain1/1  "<vcabc>"
  Unit Delay/1 -> Demux/1
  [m_filter] -> Bus Selector/1
  "abc -> dq (Power-Invariant)2"/1(dq) -> [il_dq]
  "abc -> dq (Power-Invariant)4"/1(dq) -> [ig_dq]
  "abc -> dq (Power-Invariant)1"/1(dq) -> [vc_dq]
  [vc_abc] -> "PLL (vabc -> vq)"/1(vabc)
  [il_dq] -> Current Controller/2(iIdq)
  [ig_dq] -> PQ Calculation (dq-Frame)1/2(idq)
  PQ Calculation (dq-Frame)1/1(pq) -> Scope2/1, [pq]
  [vc_dq] -> PQ Calculation (dq-Frame)1/1(vdq)
  [theta] -> "dq -> abc (Power-Invariant)1"/2(theta)
  [vc_dq] -> Current Controller/3(vdq)
  Constant/1 -> Current Controller/4(enable)
  "PLL (vabc -> vq)"/1(w) -> [w]
  "PLL (vabc -> vq)"/2(theta) -> [theta]
  Bus Selector/2 -> Gain2/1  "<ilabc>"
  Bus Selector/3 -> Gain3/1  "<igabc>"
  [theta] -> "abc -> dq (Power-Invariant)4"/2(theta)
  [ig_abc] -> "abc -> dq (Power-Invariant)4"/1(abc)
  [il_abc] -> "abc -> dq (Power-Invariant)2"/1(abc)
  [vc_abc] -> "abc -> dq (Power-Invariant)1"/1(abc)
  [theta] -> "abc -> dq (Power-Invariant)2"/2(theta)
  [theta] -> "abc -> dq (Power-Invariant)1"/2(theta)
  Demux/3 -> vc/1
  Demux/2 -> vb/1
  Demux/1 -> va/1
  LCL Filter/1(m) -> [m_filter]
  Bus Creator3/1 -> m/1
  "dq -> abc (Power-Invariant)1"/1(abc) -> Scope10/2, Saturation/1
  Vdc/1 -> [Vdc]
  P_dc/1 -> Divide/1
  [Vdc] -> Divide/2
  Divide/1 -> Scope/1, [iin]
  [iin] -> Unit Delay1/1
  [pq_converter] -> Demux1/1  "pq"
  [il_dq] -> PQ Calculation (dq-Frame)3/2(idq), PQ Calculation (dq-Frame)2/2(idq)
  PQ Calculation (dq-Frame)2/1(pq) -> Demux2/1, [pq_converter]
  Demux1/1 -> Scope1/1, Divide1/1
  [Vdc] -> Divide1/2
  Divide1/1 -> Scope1/2, [iout]
  [iout] -> Unit Delay2/1
  Voltage Controller/1(id*) -> Mux/1
  Mux/1 -> [ildq_ref], Current Controller/1(iIdq*)
  Constant2/1 -> Voltage Controller/3(enable)
  [Vdc] -> Voltage Controller/4(v_dc)
  Constant3/1 -> Voltage Controller/1(v_dc*)
  Constant4/1 -> Voltage Controller/2(id0)
  [ildq_ref] -> Bus Creator3/12  "ildq_ref"
  [Vdc] -> Bus Creator3/13  "Vdc"
  Unit Delay1/1 -> Controlled Current Source1/1
  Unit Delay2/1 -> Controlled Current Source/1
  Ug/1 -> Gain5/1
  [theta] -> "abc -> dq (Power-Invariant)3"/2(theta)
  "abc -> dq (Power-Invariant)3"/1(dq) -> Scope5/1, [Ug_dq]
  [vi_dq] -> PQ Calculation (dq-Frame)2/1(vdq)
  [Ug_dq] -> PQ Calculation (dq-Frame)3/1(vdq)
  PQ Calculation (dq-Frame)3/1(pq) -> Demux3/1
  Mux1/1 -> Scope4/1
  Demux2/1 -> Mux1/1
  Demux3/1 -> Mux1/2
  Mux2/1 -> Scope4/2
  Demux2/2 -> Mux2/1
  Demux3/2 -> Mux2/2
  Gain5/1 -> "abc -> dq (Power-Invariant)3"/1(abc)
  Constant5/1 -> Ierror/2
  Constant7/1 -> Product/2
  Product/1 -> Mux/2, Scope6/1
  [vc_dq] -> u/1
  u/1 -> Scope8/1, Ierror/1
  Ierror/1 -> Scope7/1, Filter p/1
  Filter p/1 -> Scope7/2, Product/1
  Current Controller/1(vidq*) -> Scope3/1, [vi_dq], "dq -> abc (Power-Invariant)1"/1(dq)
  Saturation/1 -> Scope10/1, [vi_abc]
  connections:
  LCL Filter/LConn3 -- vc/RConn1
  va/LConn1 -- vb/LConn1 -- vc/LConn1 -- LCL Filter/LConn4 -- N/RConn1
  LCL Filter/RConn3 -- c/RConn1
  LCL Filter/RConn2 -- b/RConn1
  LCL Filter/RConn1 -- a/RConn1
  LCL Filter/LConn1 -- va/RConn1
  LCL Filter/LConn2 -- vb/RConn1
  Vdc/LConn1 -- Controlled Current Source/LConn1 -- Controlled Current Source1/RConn1 -- Series RLC Branch/LConn1
  Controlled Current Source1/LConn1 -- Controlled Current Source/RConn1 -- Vdc/LConn2 -- Series RLC Branch/RConn1

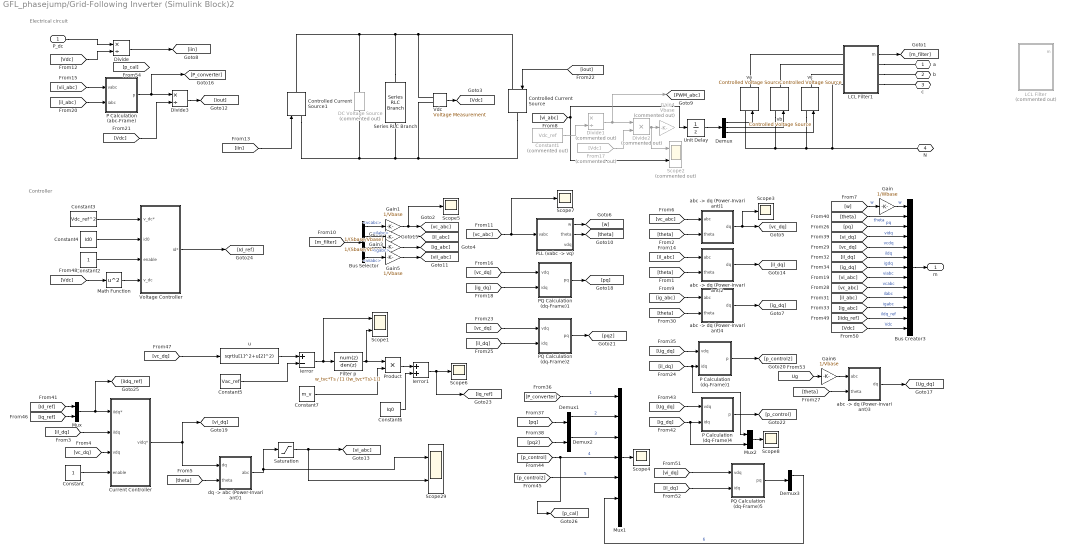
== system GFL_phasejump/Grid-Following Inverter (Simulink Block)2 ==
  note: Electrical circuit
  note: Controller
  P_dc : Inport
  Bus Creator3 : BusCreator  Inputs=13
  Bus Selector : BusSelector  OutputSignals=vcabc,ilabc,igabc,viiabc
  Constant : Constant
  Constant1 : Constant  Commented=on  Value=Vdc_ref
  Constant2 : Constant
  Constant3 : Constant  Value=Vdc_ref^2
  Constant4 : Constant  Value=Id0
  Constant5 : Constant  Value=Vac_ref
  Constant6 : Constant  Value=Iq0
  Constant7 : Constant  Value=m_v
  Controlled Current Source : spsControlledCurrentSourceLib/Controlled Current Source  Initialize=on  Source_Type=AC  Amplitude=0  Phase=0  Frequency=0  Measurements=None
  Controlled Current Source1 : spsControlledCurrentSourceLib/Controlled Current Source  Initialize=on  Source_Type=AC  Amplitude=0  Phase=0  Frequency=0  Measurements=None
  Current Controller : Subsystem  mask{Ts=Ts, Wbase=Wbase, Lf=Lf/Wbase, Kg=0, Kp=w_i*Lf/Wbase, Ki=w_i*w_i/4*Lf/Wbase, vdmax=inf, vqmax=inf, Kcd=0}
      mask prompts: Ts "Sampling Time (s)"; Wbase "Base Angular Frequency (rad/s)"; Lf "Inductance"; Kg "Estimator Gain"; Kp "Proportional Gain"; Ki "Integral Gain"; vdmax "Voltage D Limit"; vqmax "Voltage Q Limit"; Kcd "Cross Decoupling Gain"
  DC Voltage Source : spsDCVoltageSourceLib/DC Voltage Source  Commented=on  Amplitude=Vdc_ref  Measurements=None
  Demux : Demux  Outputs=3
  Demux1 : Demux  Outputs=2
  Demux2 : Demux  Outputs=2
  Demux3 : Demux  Outputs=2
  Divide : Product  Inputs=*/
  Divide1 : Product  Commented=on  Inputs=*/
  Divide2 : Product  Commented=on  Inputs=**
  Divide3 : Product  Inputs=*/
  Filter p : DiscreteTransferFcn  Numerator=w_tvc*Ts  Denominator=[1 ((w_tvc*Ts)-1)]  SampleTime=Ts
  From17 : From  Commented=on  GotoTag=Vdc
      settings: CloseFcn=tagdialog Close
  Gain : Gain  Gain=1/Wbase
  Gain1 : Gain  Gain=1/Vbase
  Gain2 : Gain  Gain=1/(Sbase/Vbase)
  Gain3 : Gain  Gain=1/(Sbase/Vbase)
  Gain4 : Gain  Commented=on  Gain=Vbase
  Gain5 : Gain  Gain=1/Vbase
  Gain6 : Gain  Gain=1/Vbase
  Ierror : Sum  Inputs=+-
  Ierror1 : Sum
  LCL Filter : Subsystem  Commented=on  mask{Lf=Lf*(Vbase^2/Sbase)/Wbase, Rf=Lf*(Vbase^2/Sbase)*1e-3, Lc=Lc*(Vbase^2/Sbase)/Wbase, Rc=Lc*(Vbase^2/Sbase)*2e-2, Cf=Cf*(Sbase/Vbase^2)/Wbase, Rd=1e-5*(Vbase^2/Sbase)}
      mask prompts: Lf "Lf (H)"; Rf "Rf (Ohm)"; Lc "Lc (H)"; Rc "Rc (Ohm)"; Cf "Cf (F)"; Rd "Rd (Ohm)"
  LCL Filter1 : Subsystem  AncestorBlock=SimplexPS/LCL Filter  mask{Lf=Lf*(Vbase^2/Sbase)/Wbase, Rf=Lf*(Vbase^2/Sbase)*2e-6, Lc=Lc*(Vbase^2/Sbase)/Wbase, Rc=Lc*(Vbase^2/Sbase)*2e-6, Cf=Cf*(Sbase/Vbase^2)/Wbase, Rd=1e-5*(Vbase^2/Sbase)}
      mask prompts: Lf "Lf (H)"; Rf "Rf (Ohm)"; Lc "Lc (H)"; Rc "Rc (Ohm)"; Cf "Cf (F)"; Rd "Rd (Ohm)"
  Math Function : Math  Operator=square
  Mux : Mux  Inputs=2
  Mux1 : Mux  Inputs=7
  Mux2 : Mux  Inputs=2
  P Calculation (abc-Frame) : Subsystem
  P Calculation (dq-Frame)1 : Subsystem
  P Calculation (dq-Frame)4 : Subsystem
  "PLL (vabc -> vq)" : Subsystem  mask{Ts=Ts, Vbase=Vbase, Wbase=Wbase, kp=kp_pll, ki=ki_pll, w_tau=w_tau, theta0=0}
      mask prompts: Ts "Ts (s), sampling period"; Vbase "Vbase (V), base voltage"; Wbase "Wbase (rad/s), base angular frequency"; kp "PLL Proportional Gain"; ki "PLL Integral Gain"; w_tau "w_tau (rad/s), low-pass filter bandwidth"; theta0 "theta0 (rad), initial angle"
  PQ Calculation (dq-Frame)1 : Subsystem
  PQ Calculation (dq-Frame)2 : Subsystem
  PQ Calculation (dq-Frame)5 : Subsystem  AncestorBlock=|
      | SimplusGT/PQ Calculation
      | (dq-Frame)
  Product : Product
  Saturation : Saturate  UpperLimit=5*sqrt(3/2) %dc_ref/sqrt(3) %5*sqrt(3/2) %  LowerLimit=-5*sqrt(3/2) %Vdc_ref/sqrt(3) %5*sqrt(3/2) %  LinearizeAsGain=off
  Scope1 : Scope  NumInputPorts=2
  Scope2 : Scope  Commented=on  NumInputPorts=2
  Scope29 : Scope  NumInputPorts=2
  Scope{3..8} (6 alike) : Scope
  Series RLC Branch : spsSeriesRLCBranchLib/Series RLC Branch  LConnTagsString=__new0  RConnTagsString=__new0  BranchType=RC  Resistance=1e-6*(Vbase^2/Sbase)  Inductance=1e-3  SetiL0=off  InitialCurrent=0  Capacitance=Y_dc*(Sbase/Vbase^2)/Wbase  Setx0=on  InitialVoltage=Vdc_ref  Measurements=None
  Unit Delay : UnitDelay  SampleTime=-1  HasFrameUpgradeWarning=on
  Vdc : spsVoltageMeasurementLib/Voltage Measurement  PhasorSimulation=off  OutputType=Complex  PSBequivalent=0
  Voltage Controller : Subsystem  mask{Ts=Ts, Kp=kp_v_dc, Ki=ki_v_dc, max=Id_limit}
      mask prompts: Ts "Sampling Time (s)"; Kp "Proportional Gain"; Ki "Integral Gain"; max "Output Limit"
  "abc -> dq (Power-Invariant)1" : Subsystem
  "abc -> dq (Power-Invariant)2" : Subsystem
  "abc -> dq (Power-Invariant)3" : Subsystem  AncestorBlock=|
      | SimplusGT/abc -> dq
      | (Power-Invariant)
  "abc -> dq (Power-Invariant)4" : Subsystem
  "dq -> abc (Power-Invariant)1" : Subsystem
  u : Fcn  Expr=sqrt(u[1]^2+u[2]^2)
  va : spsControlledVoltageSourceLib/Controlled Voltage Source  Initialize=on  Source_Type=AC  Amplitude=0  Phase=0  Frequency=0  Measurements=None
  vb : spsControlledVoltageSourceLib/Controlled Voltage Source  Initialize=on  Source_Type=AC  Amplitude=0  Phase=0  Frequency=0  Measurements=None
  vc : spsControlledVoltageSourceLib/Controlled Voltage Source  Initialize=on  Source_Type=AC  Amplitude=0  Phase=0  Frequency=0  Measurements=None
  a : PMIOPort  Side=Right
  b : PMIOPort  Port=2  Side=Right
  c : PMIOPort  Port=3  Side=Right
  N : PMIOPort  Port=4  Side=Right
  m : Outport
  wires:
  Gain3/1 -> [ig_abc]
  Gain2/1 -> [il_abc]
  Gain1/1 -> Scope5/1, [vc_abc]
  [ig_abc] -> Bus Creator3/11  "igabc"
  [il_abc] -> Bus Creator3/10  "ilabc"
  [vc_abc] -> Bus Creator3/9  "vcabc"
  [vi_abc] -> Bus Creator3/8  "viabc"
  [ig_dq] -> Bus Creator3/7  "igdq"
  [il_dq] -> Bus Creator3/6  "ildq"
  [vc_dq] -> Bus Creator3/5  "vcdq"
  [vi_dq] -> Bus Creator3/4  "vidq"
  [pq] -> Bus Creator3/3  "pq"
  [theta] -> Bus Creator3/2  "theta"
  Gain/1 -> Bus Creator3/1  "w"
  [w] -> Gain/1  "w"
  Bus Selector/1 -> Gain1/1  "<vcabc>"
  Unit Delay/1 -> Demux/1
  [m_filter] -> Bus Selector/1
  "abc -> dq (Power-Invariant)2"/1(dq) -> [il_dq]
  "abc -> dq (Power-Invariant)4"/1(dq) -> [ig_dq]
  "abc -> dq (Power-Invariant)1"/1(dq) -> Scope3/1, [vc_dq]
  [vc_abc] -> Scope7/1, "PLL (vabc -> vq)"/1(vabc)
  Mux/1 -> [iIdq_ref], Current Controller/1(iIdq*)
  [ig_dq] -> PQ Calculation (dq-Frame)1/2(idq)
  PQ Calculation (dq-Frame)1/1(pq) -> [pq]
  [vc_dq] -> PQ Calculation (dq-Frame)1/1(vdq)
  [theta] -> "dq -> abc (Power-Invariant)1"/2(theta)
  Current Controller/1(vidq*) -> "dq -> abc (Power-Invariant)1"/1(dq), [vi_dq]
  [vc_dq] -> Current Controller/3(vdq)
  Constant/1 -> Current Controller/4(enable)
  "PLL (vabc -> vq)"/1(w) -> [w]
  "PLL (vabc -> vq)"/2(theta) -> [theta]
  Bus Selector/2 -> Gain2/1  "<ilabc>"
  Bus Selector/3 -> Gain3/1  "<igabc>"
  [theta] -> "abc -> dq (Power-Invariant)4"/2(theta)
  [ig_abc] -> "abc -> dq (Power-Invariant)4"/1(abc)
  [il_abc] -> "abc -> dq (Power-Invariant)2"/1(abc)
  [vc_abc] -> "abc -> dq (Power-Invariant)1"/1(abc)
  [theta] -> "abc -> dq (Power-Invariant)2"/2(theta)
  [theta] -> "abc -> dq (Power-Invariant)1"/2(theta)
  Demux/3 -> vc/1
  Demux/2 -> vb/1
  Demux/1 -> va/1
  LCL Filter1/1(m) -> [m_filter]
  Bus Creator3/1 -> m/1
  "dq -> abc (Power-Invariant)1"/1(abc) -> Saturation/1, Scope29/1
  Saturation/1 -> [vi_abc], Scope29/2
  [il_dq] -> Current Controller/2(iIdq)
  [iout] -> Controlled Current Source/1
  [iin] -> Controlled Current Source1/1
  Vdc/1 -> [Vdc]
  Divide/1 -> [iin]
  [Vdc] -> Divide/2
  P_dc/1 -> Divide/1
  [vi_abc] -> Scope2/2, Unit Delay/1
  Divide2/1 -> Scope2/1, Gain4/1
  Divide1/1 -> [PWM_abc], Divide2/1
  Constant1/1 -> Divide1/2
  From17/1 -> Divide2/2
  [vii_abc] -> P Calculation (abc-Frame)/1(vabc)
  Bus Selector/4 -> Gain5/1  "<viiabc>"
  Gain5/1 -> [vii_abc]
  [il_abc] -> P Calculation (abc-Frame)/2(iabc)
  [Vdc] -> Divide3/2
  Divide3/1 -> [iout]
  [Ug_dq] -> P Calculation (dq-Frame)1/1(vdq)
  [il_dq] -> Mux2/1, P Calculation (dq-Frame)1/2(idq)
  Gain6/1 -> "abc -> dq (Power-Invariant)3"/1(abc)
  "abc -> dq (Power-Invariant)3"/1(dq) -> [Ug_dq]
  [Ug] -> Gain6/1
  [theta] -> "abc -> dq (Power-Invariant)3"/2(theta)
  P Calculation (dq-Frame)1/1(p) -> [p_control2]
  [il_dq] -> PQ Calculation (dq-Frame)2/2(idq)
  [vc_dq] -> PQ Calculation (dq-Frame)2/1(vdq)
  PQ Calculation (dq-Frame)2/1(pq) -> [pq2]
  [pq] -> Demux1/1
  [pq2] -> Demux2/1
  [ig_dq] -> Mux2/2, P Calculation (dq-Frame)4/2(idq)
  [Ug_dq] -> P Calculation (dq-Frame)4/1(vdq)
  P Calculation (dq-Frame)4/1(p) -> [p_control]
  [P_converter] -> Mux1/1  "1"
  Demux1/1 -> Mux1/2  "2"
  Demux2/1 -> Mux1/3  "3"
  [p_control] -> [p_cal], Mux1/4  "4"
  [p_control2] -> Mux1/5  "5"
  [Id_ref] -> Mux/1
  [Iq_ref] -> Mux/2
  u/1 -> Ierror/1
  Ierror/1 -> Scope1/1, Filter p/1
  Filter p/1 -> Scope1/2, Product/1
  [vc_dq] -> u/1
  Constant7/1 -> Product/2
  Constant5/1 -> Ierror/2
  Constant2/1 -> Voltage Controller/3(enable)
  [Vdc] -> Math Function/1
  Constant3/1 -> Voltage Controller/1(v_dc*)
  Constant4/1 -> Voltage Controller/2(id0)
  [iIdq_ref] -> Bus Creator3/12  "ildq_ref"
  [Vdc] -> Bus Creator3/13  "Vdc"
  [vi_dq] -> PQ Calculation (dq-Frame)5/1(vdq)
  [il_dq] -> PQ Calculation (dq-Frame)5/2(idq)
  PQ Calculation (dq-Frame)5/1(pq) -> Demux3/1
  Demux3/1 -> Mux1/6  "6"
  Voltage Controller/1(id*) -> [Id_ref]
  Mux1/1 -> Scope4/1
  Math Function/1 -> Voltage Controller/4(v_dc)
  Mux2/1 -> Scope8/1
  P Calculation (abc-Frame)/1(p) -> Divide3/1, [P_converter]
  Product/1 -> Ierror1/1
  Ierror1/1 -> [Iq_ref], Scope6/1
  Constant6/1 -> Ierror1/2
  connections:
  LCL Filter1/LConn3 -- vc/RConn1
  va/LConn1 -- vb/LConn1 -- vc/LConn1 -- N/RConn1 -- LCL Filter1/LConn4
  LCL Filter1/RConn3 -- c/RConn1
  LCL Filter1/RConn2 -- b/RConn1
  LCL Filter1/RConn1 -- a/RConn1
  LCL Filter1/LConn1 -- va/RConn1
  LCL Filter1/LConn2 -- vb/RConn1
  Controlled Current Source1/LConn1 -- Series RLC Branch/RConn1 -- Controlled Current Source/RConn1 -- Vdc/LConn2 -- DC Voltage Source/LConn1
  Series RLC Branch/LConn1 -- Vdc/LConn1 -- Controlled Current Source/LConn1 -- Controlled Current Source1/RConn1 -- DC Voltage Source/RConn1

== system GFL_phasejump/Single Sag2 ==
  note: Pulse generator
      |
      | Author(s): Yitong Li
  Constant : Constant
  Gain : Gain  Gain=1-Am
  Product : Product
  Step : Step  Time=t0  SampleTime=0
  Step1 : Step  Time=t0+dt  Before=1  After=0  SampleTime=0
  Subtract : Sum  Inputs=+-
  Out : Outport
  wires:
  Step1/1 -> Product/2
  Step/1 -> Product/1
  Product/1 -> Gain/1
  Gain/1 -> Subtract/2
  Subtract/1 -> Out/1
  Constant/1 -> Subtract/1

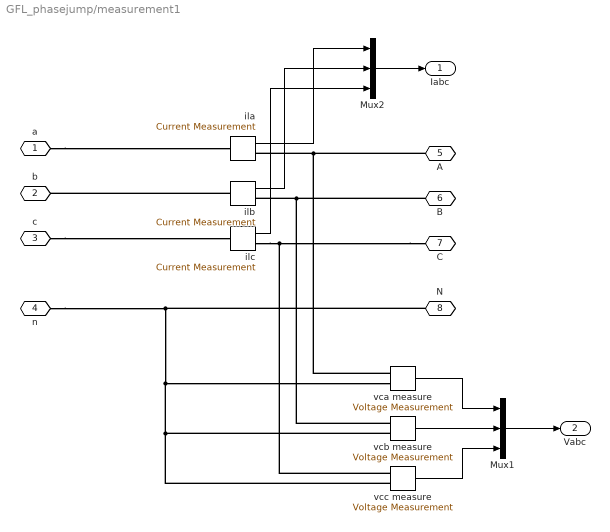
== system GFL_phasejump/measurement1 ==
  Mux1 : Mux  Inputs=3
  Mux2 : Mux  Inputs=3
  ila : spsCurrentMeasurementLib/Current Measurement  PhasorSimulation=off  OutputType=Complex  PSBequivalent=0
  ilb : spsCurrentMeasurementLib/Current Measurement  PhasorSimulation=off  OutputType=Complex  PSBequivalent=0
  ilc : spsCurrentMeasurementLib/Current Measurement  PhasorSimulation=off  OutputType=Complex  PSBequivalent=0
  vca measure : spsVoltageMeasurementLib/Voltage Measurement  PhasorSimulation=off  OutputType=Complex  PSBequivalent=0
  vcb measure : spsVoltageMeasurementLib/Voltage Measurement  PhasorSimulation=off  OutputType=Complex  PSBequivalent=0
  vcc measure : spsVoltageMeasurementLib/Voltage Measurement  PhasorSimulation=off  OutputType=Complex  PSBequivalent=0
  a : PMIOPort  Side=Left
  b : PMIOPort  Port=2  Side=Left
  c : PMIOPort  Port=3  Side=Left
  n : PMIOPort  Port=4  Side=Left
  A : PMIOPort  Port=5  Side=Right
  B : PMIOPort  Port=6  Side=Right
  C : PMIOPort  Port=7  Side=Right
  N : PMIOPort  Port=8  Side=Right
  Iabc : Outport
  Vabc : Outport  Port=2
  wires:
  ila/1 -> Mux2/1
  ilb/1 -> Mux2/2
  ilc/1 -> Mux2/3
  Mux2/1 -> Iabc/1
  vcb measure/1 -> Mux1/2
  vca measure/1 -> Mux1/1
  vcc measure/1 -> Mux1/3
  Mux1/1 -> Vabc/1
  connections:
  a/RConn1 -- ila/LConn1
  ila/RConn1 -- A/RConn1 -- vca measure/LConn1
  ilb/LConn1 -- b/RConn1
  ilb/RConn1 -- B/RConn1 -- vcb measure/LConn1
  c/RConn1 -- ilc/LConn1
  C/RConn1 -- ilc/RConn1 -- vcc measure/LConn1
  n/RConn1 -- vcc measure/LConn2 -- vcb measure/LConn2 -- vca measure/LConn2 -- N/RConn1

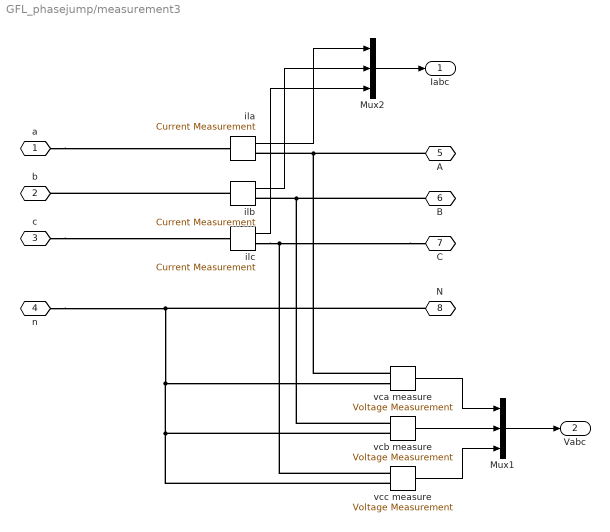
== system GFL_phasejump/measurement3 ==
  Mux1 : Mux  Inputs=3
  Mux2 : Mux  Inputs=3
  ila : spsCurrentMeasurementLib/Current Measurement  PhasorSimulation=off  OutputType=Complex  PSBequivalent=0
  ilb : spsCurrentMeasurementLib/Current Measurement  PhasorSimulation=off  OutputType=Complex  PSBequivalent=0
  ilc : spsCurrentMeasurementLib/Current Measurement  PhasorSimulation=off  OutputType=Complex  PSBequivalent=0
  vca measure : spsVoltageMeasurementLib/Voltage Measurement  PhasorSimulation=off  OutputType=Complex  PSBequivalent=0
  vcb measure : spsVoltageMeasurementLib/Voltage Measurement  PhasorSimulation=off  OutputType=Complex  PSBequivalent=0
  vcc measure : spsVoltageMeasurementLib/Voltage Measurement  PhasorSimulation=off  OutputType=Complex  PSBequivalent=0
  a : PMIOPort  Side=Left
  b : PMIOPort  Port=2  Side=Left
  c : PMIOPort  Port=3  Side=Left
  n : PMIOPort  Port=4  Side=Left
  A : PMIOPort  Port=5  Side=Right
  B : PMIOPort  Port=6  Side=Right
  C : PMIOPort  Port=7  Side=Right
  N : PMIOPort  Port=8  Side=Right
  Iabc : Outport
  Vabc : Outport  Port=2
  wires:
  ila/1 -> Mux2/1
  ilb/1 -> Mux2/2
  ilc/1 -> Mux2/3
  Mux2/1 -> Iabc/1
  vcb measure/1 -> Mux1/2
  vca measure/1 -> Mux1/1
  vcc measure/1 -> Mux1/3
  Mux1/1 -> Vabc/1
  connections:
  a/RConn1 -- ila/LConn1
  ila/RConn1 -- A/RConn1 -- vca measure/LConn1
  ilb/LConn1 -- b/RConn1
  ilb/RConn1 -- B/RConn1 -- vcb measure/LConn1
  c/RConn1 -- ilc/LConn1
  C/RConn1 -- ilc/RConn1 -- vcc measure/LConn1
  n/RConn1 -- vcc measure/LConn2 -- vcb measure/LConn2 -- vca measure/LConn2 -- N/RConn1
